simulink model "PHIL_voltage_source_set"  (R2016a)
settings: Solver=FixedStepDiscrete  SolverMode=SingleTasking  StartTime=0.0  StopTime=2  FixedStep=2e-4  RelTol=1e-3
settings Model: Creator=CoSES_HPC2  LastModifiedBy=CoSES_HPC2
settings DataIOCC: ReturnWorkspaceOutputs=on
settings DebuggingCC: RootOutportRequireBusObject=error  StrictBusMsg=ErrorOnBusTreatedAsVector  SFUnexpectedBacktrackingDiag=error  SFNoUnconditionalDefaultTransitionDiag=error
settings HardwareCC: ProdBitPerPointer=32  ProdLargestAtomicFloat=None  ProdWordSize=32  ProdHWDeviceType=Intel->x86/Pentium
settings SFSimCC: SimUseLocalCustomCode=on
settings RTWCC: SystemTargetFile=NIVeriStand.tlc  TemplateMakefile=NIVeriStand_vc.tmf  Description=NI Phar Lap Real-Time & Windows Targets  RTWUseLocalCustomCode=on
settings STFCustomTargetCC: MatFileLogging=on  SystemTargetFile=NIVeriStand.tlc
settings GRTTargetCC: ParMdlRefBuildCompliant=off  CompOptLevelCompliant=off  ConcurrentExecutionCompliant=off  GeneratePreprocessorConditionals=Use local settings  CombineOutputUpdateFcns=off  CPPClassGenCompliant=off  GRTInterface=on  UseToolchainInfoCompliant=off
settings ConfigComp: CovMetricSettings=dwe  CovHtmlReporting=off  CovSaveCumulativeToWorkspaceVar=off  CovSaveSingleToWorkspaceVar=off  CovExternalEMLEnable=on

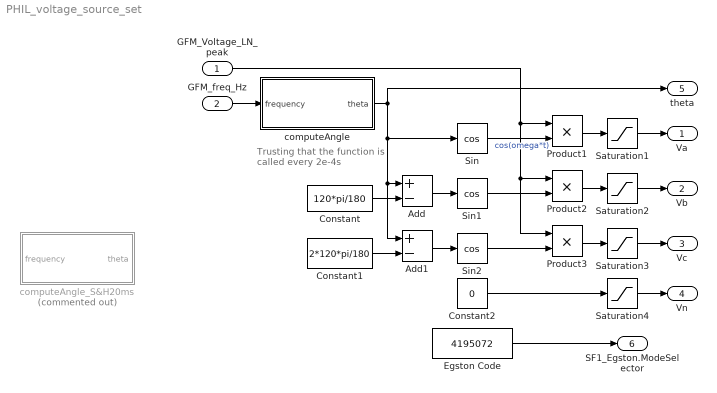
== system PHIL_voltage_source_set ==
  note: Trusting that the function
      | is called every 2e-4s
  GFM_Voltage_LN_peak : Inport
  GFM_freq_Hz : Inport  Port=2  Interpolate=off
  Add : Sum  Inputs=+-
  Add1 : Sum  Inputs=+-
  Constant : Constant  Value=120*pi/180
  Constant1 : Constant  Value=2*120*pi/180
  Constant2 : Constant  Value=0
  Egston Code : Constant  Value=4195072
  Product1 : Product
  Product2 : Product
  Product3 : Product
  Saturation{1..4} (4 alike) : Saturate  UpperLimit=400  LowerLimit=-400
  Sin : Trigonometry  Operator=cos  ApproximationMethod=CORDIC  OutputSignalType=real
  Sin1 : Trigonometry  Operator=cos  ApproximationMethod=CORDIC  OutputSignalType=real
  Sin2 : Trigonometry  Operator=cos  ApproximationMethod=CORDIC  OutputSignalType=real
  computeAngle : MATLAB Function  TreatAsAtomicUnit=on
  computeAngle_S&H20ms : MATLAB Function  Commented=on  TreatAsAtomicUnit=on
  Va : Outport
  Vb : Outport  Port=2
  Vc : Outport  Port=3
  Vn : Outport  Port=4
  theta : Outport  Port=5
  SF1_Egston.ModeSelector : Outport  Port=6
  wires:
  Sin/1 -> Product1/2  "cos(omega*t)"
  Product1/1 -> Saturation1/1
  Add/1 -> Sin1/1
  Constant/1 -> Add/2
  Add1/1 -> Sin2/1
  Constant1/1 -> Add1/2
  Sin1/1 -> Product2/2
  Sin2/1 -> Product3/2
  Product2/1 -> Saturation2/1
  Product3/1 -> Saturation3/1
  Constant2/1 -> Saturation4/1
  Saturation1/1 -> Va/1
  Saturation2/1 -> Vb/1
  Saturation3/1 -> Vc/1
  Saturation4/1 -> Vn/1
  GFM_Voltage_LN_peak/1 -> Product1/1, Product3/1, Product2/1
  computeAngle/1(theta) -> Add1/1, Add/1, Sin/1, theta/1
  GFM_freq_Hz/1 -> computeAngle/1(frequency)
  Egston Code/1 -> SF1_Egston.ModeSelector/1

== matlab function PHIL_voltage_source_set/computeAngle_S&H20ms ==
  data: frequency input; theta output
function theta = computeAngle(frequency)
    % Define persistent variables to hold state between function calls
    persistent lastFrequency;
    persistent cumulativeTheta;
    persistent sampleCounter;

    % Define the sample time (20 ms)
    sampleTime = 20e-3; % seconds
    callTime = 2e-4;    % seconds (function call time)

    % Initialize persistent variables on the first call
    if isempty(lastFrequency)
        lastFrequency = frequency; % Initialize with the first frequency
        cumulativeTheta = 0;       % Initialize cumulative angle
        sampleCounter = 0;         % Initialize sample counter
    end

    % Increment the sample counter
    sampleCounter = sampleCounter + callTime;

    % Sample the frequency every 20 ms
    if sampleCounter >= sampleTime
        lastFrequency = frequency; % Update the last frequency
        sampleCounter = 0;         % Reset the sample counter
    end

    % Calculate the angular increment (deltaTheta)
    deltaTheta = 2 * pi * lastFrequency * callTime;

    % Update the cumulative angle
    cumulativeTheta = cumulativeTheta + deltaTheta;

    % Apply modulo to keep theta within [0, 2*pi]
    theta = mod(cumulativeTheta, 2 * pi);
end

== matlab function PHIL_voltage_source_set/computeAngle ==
  data: frequency input; theta output
function theta = computeAngle(frequency)
    % Define persistent variables to hold state between function calls
    persistent cumulativeTheta;

    % Define the time step used in the settings
    dt = 2e-4; % seconds (function call time)

    % Initialize persistent variables on the first call
    if isempty(cumulativeTheta)
        cumulativeTheta = 0; % Initialize cumulative angle
    end

    % Compute the amount of growth in theta during this time step
    deltaTheta = (2 * pi * frequency * dt);

    % Update the cumulative angle
    cumulativeTheta = cumulativeTheta + deltaTheta;

    % Apply modulo to keep theta within [0, 2*pi)
    theta = mod(cumulativeTheta, 2 * pi);
end
